simulink model "SignatureDemo_STRONG_SIGNATURE1"  (Simulink 7.8)
settings: Solver=ode3  StartTime=0.0  StopTime=10.0  RelTol=1e-3
settings Model: Creator=Jeff  LastModifiedBy=Ben

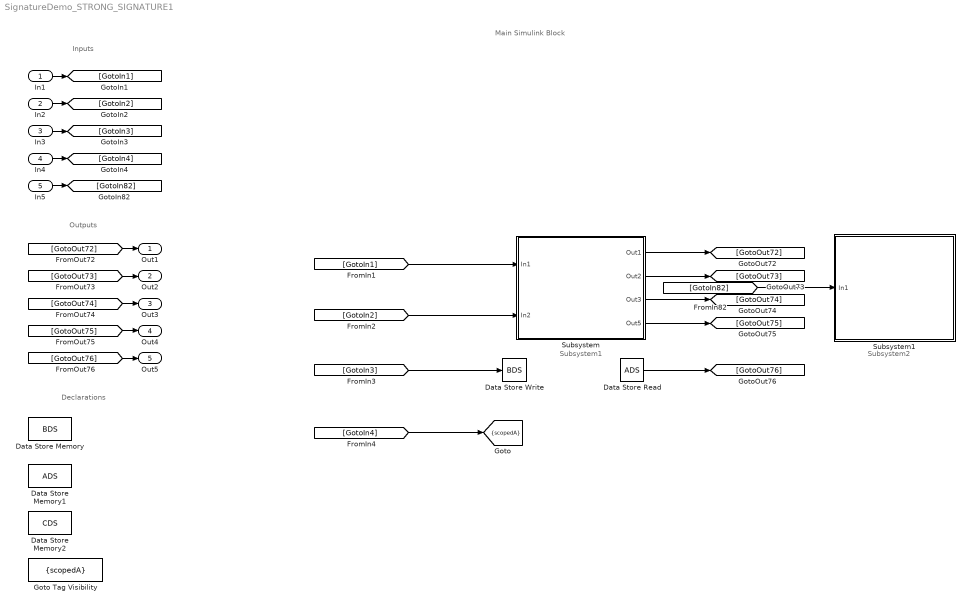
== system SignatureDemo_STRONG_SIGNATURE1 ==
  note: Subsystem1
  note: Subsystem2
  note: Main Simulink Block
  note: Inputs
  note: Outputs
  note: Declarations
  In1 : Inport
  In2 : Inport  Port=2
  In3 : Inport  Port=3
  In4 : Inport  Port=4
  In5 : Inport  Port=5
  Data Store Memory : DataStoreMemory  DataStoreName=BDS  ReadBeforeWriteMsg=warning  WriteAfterWriteMsg=warning  WriteAfterReadMsg=warning
  Data Store Memory1 : DataStoreMemory  DataStoreName=ADS  ReadBeforeWriteMsg=warning  WriteAfterWriteMsg=warning  WriteAfterReadMsg=warning
  Data Store Memory2 : DataStoreMemory  DataStoreName=CDS  ReadBeforeWriteMsg=warning  WriteAfterWriteMsg=warning  WriteAfterReadMsg=warning
  Data Store Read : DataStoreRead  DataStoreName=ADS
  Data Store Write : DataStoreWrite  DataStoreName=BDS
  Goto Tag Visibility : GotoTagVisibility  GotoTag=scopedA
  Subsystem : Subsystem
  Subsystem1 : Subsystem
  Out1 : Outport
  Out2 : Outport  Port=2
  Out3 : Outport  Port=3
  Out4 : Outport  Port=4
  Out5 : Outport  Port=5
  tag scope: scopedA=scoped
  wires:
  [GotoIn1] -> Subsystem/1(In1)
  In1/1 -> [GotoIn1]
  [GotoIn2] -> Subsystem/2(In2)
  In2/1 -> [GotoIn2]
  [GotoIn3] -> Data Store Write/1
  In3/1 -> [GotoIn3]
  [GotoIn4] -> [scopedA]
  In4/1 -> [GotoIn4]
  [GotoIn82] -> Subsystem1/1(In1)
  In5/1 -> [GotoIn82]
  Subsystem/1(Out1) -> [GotoOut72]
  Subsystem/2(Out2) -> [GotoOut73]
  Subsystem/3(Out3) -> [GotoOut74]
  Subsystem/4(Out5) -> [GotoOut75]
  Data Store Read/1 -> [GotoOut76]
  [GotoOut72] -> Out1/1
  [GotoOut73] -> Out2/1
  [GotoOut74] -> Out3/1
  [GotoOut75] -> Out4/1
  [GotoOut76] -> Out5/1

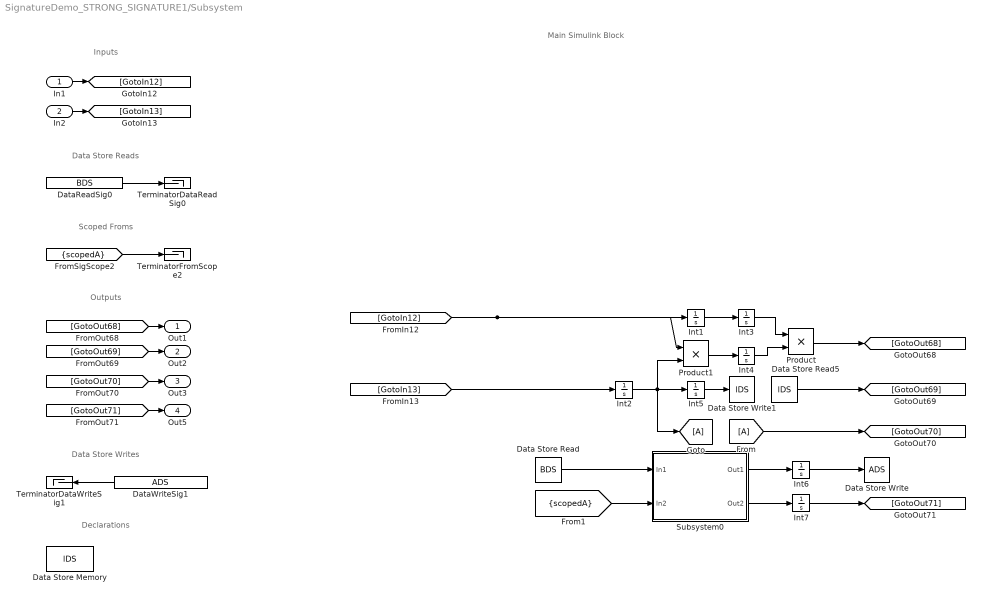
== system SignatureDemo_STRONG_SIGNATURE1/Subsystem ==
  note: Main Simulink Block
  note: Inputs
  note: Data Store Reads
  note: Scoped Froms
  note: Outputs
  note: Data Store Writes
  note: Declarations
  In1 : Inport
  In2 : Inport  Port=2
  Data Store Memory : DataStoreMemory  DataStoreName=lDS  ReadBeforeWriteMsg=warning  WriteAfterWriteMsg=warning  WriteAfterReadMsg=warning
  Data Store Read : DataStoreRead  DataStoreName=BDS
  Data Store Read5 : DataStoreRead  DataStoreName=lDS
  Data Store Write : DataStoreWrite  DataStoreName=ADS
  Data Store Write1 : DataStoreWrite  DataStoreName=lDS
  DataReadSig0 : DataStoreRead  DataStoreName=BDS
  DataWriteSig1 : DataStoreRead  DataStoreName=ADS
  Int{1..7} (7 alike) : Integrator
  Product : Product  RndMeth=Zero
  Product1 : Product  RndMeth=Zero
  Subsystem0 : Subsystem
  TerminatorDataReadSig0 : Terminator
  TerminatorDataWriteSig1 : Terminator
  TerminatorFromScope2 : Terminator
  Out1 : Outport
  Out2 : Outport  Port=2
  Out3 : Outport  Port=3
  Out5 : Outport  Port=4
  wires:
  Int1/1 -> Int3/1
  Int3/1 -> Product/1
  Int4/1 -> Product/2
  Product1/1 -> Int4/1
  Int2/1 -> Product1/2, [A], Int5/1
  Subsystem0/1(Out1) -> Int6/1
  Subsystem0/2(Out2) -> Int7/1
  [scopedA] -> Subsystem0/2(In2)
  Data Store Read/1 -> Subsystem0/1(In1)
  Int6/1 -> Data Store Write/1
  Int5/1 -> Data Store Write1/1
  [GotoIn12] -> Product1/1, Int1/1
  In1/1 -> [GotoIn12]
  [GotoIn13] -> Int2/1
  In2/1 -> [GotoIn13]
  Product/1 -> [GotoOut68]
  Data Store Read5/1 -> [GotoOut69]
  [A] -> [GotoOut70]
  Int7/1 -> [GotoOut71]
  DataReadSig0/1 -> TerminatorDataReadSig0/1
  DataWriteSig1/1 -> TerminatorDataWriteSig1/1
  [scopedA] -> TerminatorFromScope2/1
  [GotoOut68] -> Out1/1
  [GotoOut69] -> Out2/1
  [GotoOut70] -> Out3/1
  [GotoOut71] -> Out5/1

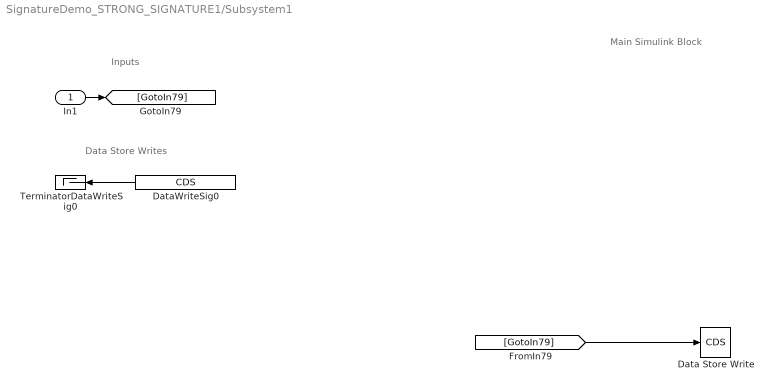
== system SignatureDemo_STRONG_SIGNATURE1/Subsystem1 ==
  note: Main Simulink Block
  note: Inputs
  note: Data Store Writes
  In1 : Inport
  Data Store Write : DataStoreWrite  DataStoreName=CDS
  DataWriteSig0 : DataStoreRead  DataStoreName=CDS
  TerminatorDataWriteSig0 : Terminator
  wires:
  [GotoIn79] -> Data Store Write/1
  In1/1 -> [GotoIn79]
  DataWriteSig0/1 -> TerminatorDataWriteSig0/1

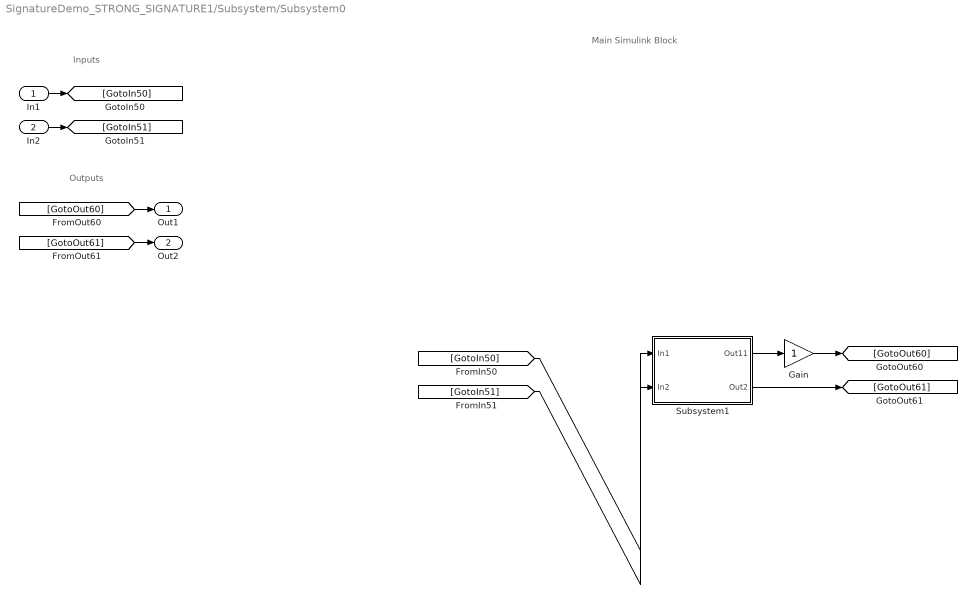
== system SignatureDemo_STRONG_SIGNATURE1/Subsystem/Subsystem0 ==
  note: Main Simulink Block
  note: Inputs
  note: Outputs
  In1 : Inport
  In2 : Inport  Port=2
  Gain : Gain
  Subsystem1 : Subsystem
  Out1 : Outport
  Out2 : Outport  Port=2
  wires:
  Subsystem1/1(Out11) -> Gain/1
  [GotoIn50] -> Subsystem1/1(In1)
  In1/1 -> [GotoIn50]
  [GotoIn51] -> Subsystem1/2(In2)
  In2/1 -> [GotoIn51]
  Gain/1 -> [GotoOut60]
  Subsystem1/2(Out2) -> [GotoOut61]
  [GotoOut60] -> Out1/1
  [GotoOut61] -> Out2/1

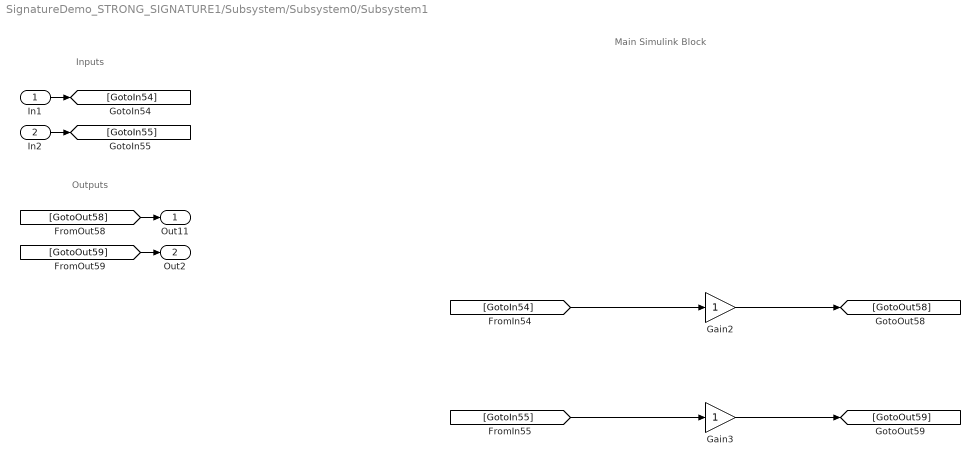
== system SignatureDemo_STRONG_SIGNATURE1/Subsystem/Subsystem0/Subsystem1 ==
  note: Main Simulink Block
  note: Inputs
  note: Outputs
  In1 : Inport
  In2 : Inport  Port=2
  Gain2 : Gain
  Gain3 : Gain
  Out11 : Outport
  Out2 : Outport  Port=2
  wires:
  [GotoIn54] -> Gain2/1
  In1/1 -> [GotoIn54]
  [GotoIn55] -> Gain3/1
  In2/1 -> [GotoIn55]
  Gain2/1 -> [GotoOut58]
  Gain3/1 -> [GotoOut59]
  [GotoOut58] -> Out11/1
  [GotoOut59] -> Out2/1
